simulink model "Battery_Model"  (R2023a)
settings: Solver=ode23tb  StartTime=0.0  StopTime=2500  FixedStep=0.1  MaxStep=0.01  MinStep=0.001  RelTol=1e-3
values from neighbouring files (symbols this model uses):
  Battery_Capacity_Ah = 3.3    [Battery_data_params.m]    (also in battery_params_v2.m = 2.4)
  Battery_SOC = linspace(0, 1, 100)    [Battery_OCV_calculation.m]    (also in Battery_data_params.m = [0	5	10	15	20	25	30	35	40	45	50	55	60	65	70	75	80	85	90	95	1; battery_params_v2.m = [0	5	10	15	20	25	30	35	40	45	50	55	60	65	70	75	80	85	90	95	1)
  Battery_SOC0 = 60    [Battery_data_params.m]    (also in battery_params_v2.m = 50)
  Cp_pack = (Nparalel*Cp)/Nserie    (= 18823.0076923)    [battery_params_v2.m]
  Rp_pack = (Nserie*Rp)/Nparalel    (= 0.001391)    [battery_params_v2.m]
  Rs_pack = (Nserie*Rs)/Nparalel    (= 0.00485124137931)    [battery_params_v2.m]
  V_pack_OCV = Nserie*Battery_U_OCV    [battery_params_v2.m]
libraries: simulink x1
settings Model: Creator=lucea  LastModifiedBy=gabrielcrisan

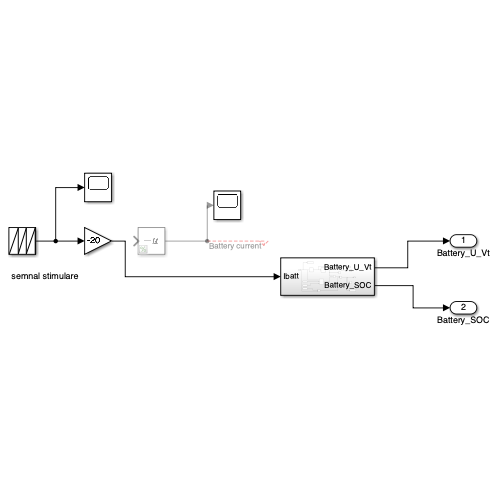
[thumbnail: Simulink's stored preview of the top-level diagram]
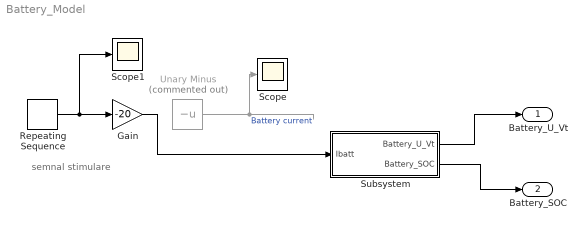
== system Battery_Model ==
  note: semnal stimulare
  Gain : Gain  Gain=-20
  Repeating Sequence : simulink/Sources/Repeating Sequence  rep_seq_t=time  rep_seq_y=pulse
  Scope : Scope
  Scope1 : Scope
  Subsystem : Subsystem
  Unary Minus : UnaryMinus  Commented=on
  Battery_U_Vt : Outport
  Battery_SOC : Outport  Port=2
  wires:
  Unary Minus/1 -> Scope/1  "Battery current"
  Subsystem/1(Battery_U_Vt) -> Battery_U_Vt/1
  Subsystem/2(Battery_SOC) -> Battery_SOC/1
  Repeating Sequence/1 -> Scope1/1, Gain/1
  Gain/1 -> Subsystem/1(Ibatt)

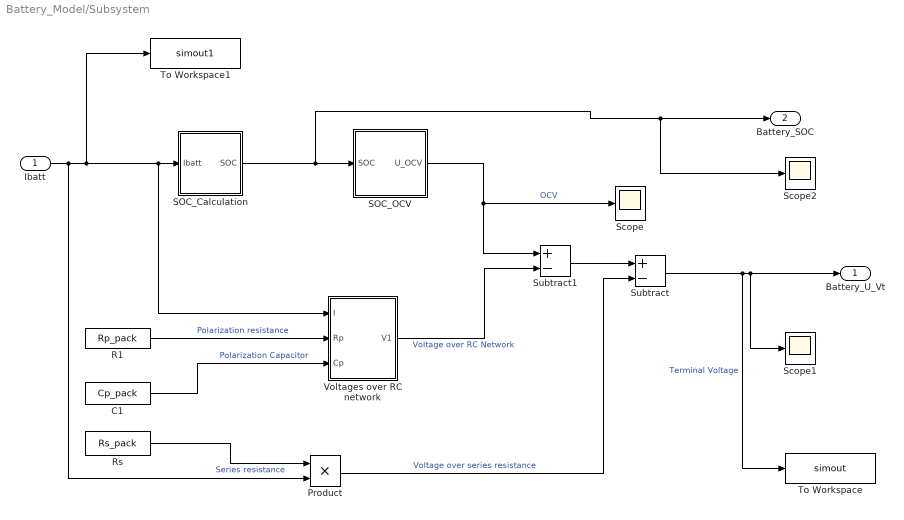
== system Battery_Model/Subsystem ==
  Ibatt : Inport
  C1 : Constant  Value=Cp_pack
  Product : Product
  R1 : Constant  Value=Rp_pack
  Rs : Constant  Value=Rs_pack
  SOC_Calculation : Subsystem
  SOC_OCV : Subsystem
  Scope : Scope
  Scope1 : Scope
  Scope2 : Scope
  Subtract : Sum  Inputs=+-
  Subtract1 : Sum  Inputs=+-
  To Workspace : ToWorkspace  VariableName=simout  SaveFormat=Timeseries  SampleTime=-1
  To Workspace1 : ToWorkspace  VariableName=simout1  SaveFormat=Timeseries  SampleTime=-1
  Voltages over RC network : Subsystem
  Battery_U_Vt : Outport
  Battery_SOC : Outport  Port=2
  wires:
  Subtract/1 -> To Workspace/1, Battery_U_Vt/1, Scope1/1  "Terminal Voltage"
  Rs/1 -> Product/1  "Series resistance"
  C1/1 -> Voltages over RC network/3(Cp)  "Polarization Capacitor"
  SOC_OCV/1(U_OCV) -> Scope/1, Subtract1/1  "OCV"
  SOC_Calculation/1(SOC) -> Scope2/1, Battery_SOC/1, SOC_OCV/1(SOC)
  Subtract1/1 -> Subtract/1
  Ibatt/1 -> Product/2, To Workspace1/1, Voltages over RC network/1(I), SOC_Calculation/1(Ibatt)
  Voltages over RC network/1(V1) -> Subtract1/2  "Voltage over RC Network"
  R1/1 -> Voltages over RC network/2(Rp)  "Polarization resistance"
  Product/1 -> Subtract/2  "Voltage over series resistance"

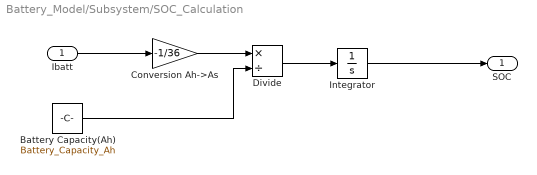
== system Battery_Model/Subsystem/SOC_Calculation ==
  Ibatt : Inport
  Battery Capacity(Ah) : Constant  Value=Battery_Capacity_Ah
  Conversion Ah->As : Gain  Gain=-1/36
  Divide : Product  Inputs=*/
  Integrator : Integrator  InitialCondition=Battery_SOC0
  SOC : Outport
  wires:
  Divide/1 -> Integrator/1
  Battery Capacity(Ah)/1 -> Divide/2
  Conversion Ah->As/1 -> Divide/1
  Ibatt/1 -> Conversion Ah->As/1
  Integrator/1 -> SOC/1

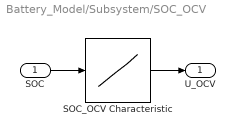
== system Battery_Model/Subsystem/SOC_OCV ==
  SOC : Inport
  SOC_OCV Characteristic : Lookup_n-D  NumberOfTableDimensions=1  BreakpointsForDimension1=Battery_SOC  Table=V_pack_OCV  InternalRulePriority=Speed  RndMeth=Simplest
  U_OCV : Outport
  wires:
  SOC/1 -> SOC_OCV Characteristic/1
  SOC_OCV Characteristic/1 -> U_OCV/1

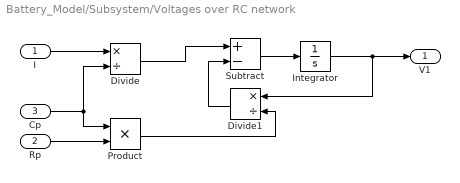
== system Battery_Model/Subsystem/Voltages over RC network ==
  I : Inport
  Rp : Inport  Port=2
  Cp : Inport  Port=3
  Divide : Product  Inputs=*/
  Divide1 : Product  Inputs=*/
  Integrator : Integrator
  Product : Product
  Subtract : Sum  Inputs=+-
  V1 : Outport
  wires:
  Rp/1 -> Product/2
  Integrator/1 -> V1/1, Divide1/1
  I/1 -> Divide/1
  Divide/1 -> Subtract/1
  Divide1/1 -> Subtract/2
  Cp/1 -> Divide/2, Product/1
  Product/1 -> Divide1/2
  Subtract/1 -> Integrator/1
